simulink model "AccPed_DrvDemLead"  (R2016b)
settings: configuration reference "CodeGenConfigSet" (kept outside this file)
values from neighbouring files (symbols this model uses):
  ACCPED_OVRRUNRMP_SY = uint8(1)    [init_AccPed_DrvDemLead.m]    (also in init_AccPed_DrvDemLead_SIL.m)
  ACCPED_REVGEARMAP_SY = uint8(1)    [init_AccPed_DrvDemLead.m]    (also in init_AccPed_DrvDemLead_SIL.m)
  AccPed_rThresPrp_C = Calibration.Parameter    [init_AccPed_DrvDemLead.m]    (also in init_AccPed_DrvDemLead_SIL.m = Simulink.Parameter)
  AccPed_rZero_C = Calibration.Parameter    [init_AccPed_DrvDemLead.m]    (also in init_AccPed_DrvDemLead_SIL.m = Simulink.Parameter)
  AccPed_trqEngRev_MAP = Calibration.Parameter    [init_AccPed_DrvDemLead.m]    (also in init_AccPed_DrvDemLead_SIL.m = Simulink.Parameter)
  AccPed_trqEngRev_MAPX = Calibration.Parameter    [init_AccPed_DrvDemLead.m]    (also in init_AccPed_DrvDemLead_SIL.m = Simulink.Parameter)
  AccPed_trqEngRev_MAPY = Calibration.Parameter    [init_AccPed_DrvDemLead.m]    (also in init_AccPed_DrvDemLead_SIL.m = Simulink.Parameter)
  AccPed_trqPrp_MAP = Calibration.Parameter    [init_AccPed_DrvDemLead.m]    (also in init_AccPed_DrvDemLead_SIL.m = Simulink.Parameter)
  AccPed_trqPrp_MAPX = Calibration.Parameter    [init_AccPed_DrvDemLead.m]    (also in init_AccPed_DrvDemLead_SIL.m = Simulink.Parameter)
  AccPed_trqPrp_MAPY = Calibration.Parameter    [init_AccPed_DrvDemLead.m]    (also in init_AccPed_DrvDemLead_SIL.m = Simulink.Parameter)
  MoFDrDem_trqEng_MAP = Calibration.Parameter    [init_AccPed_DrvDemLead.m]    (also in init_AccPed_DrvDemLead_SIL.m = Simulink.Parameter)
  MoFDrDem_trqEng_MAPX = Calibration.Parameter    [init_AccPed_DrvDemLead.m]    (also in init_AccPed_DrvDemLead_SIL.m = Simulink.Parameter)
  MoFDrDem_trqEng_MAPY = Calibration.Parameter    [init_AccPed_DrvDemLead.m]    (also in init_AccPed_DrvDemLead_SIL.m = Simulink.Parameter)
  MSTSHFT_SY = uint8(0)    [init_AccPed_DrvDemLead.m]    (also in init_AccPed_DrvDemLead_SIL.m)
  SigTst_swtAccPedLead_C = Calibration.Parameter    [init_AccPed_DrvDemLead.m]    (also in init_AccPed_DrvDemLead_SIL.m = Simulink.Parameter)
  SigTst_trqAccPedLead_C = Calibration.Parameter    [init_AccPed_DrvDemLead.m]    (also in init_AccPed_DrvDemLead_SIL.m = Simulink.Parameter)
  TRQPRPHIGH_ZERO = int16(0)    [init_AccPed_DrvDemLead.m]    (also in init_AccPed_DrvDemLead_SIL.m)
undefined symbols (not defined in the file or in its folder): Switch_conv
settings Model: Creator=lenovo  LastModifiedBy=bianxuyin
settings ConfigSetRef: SourceLocation=Base Workspace

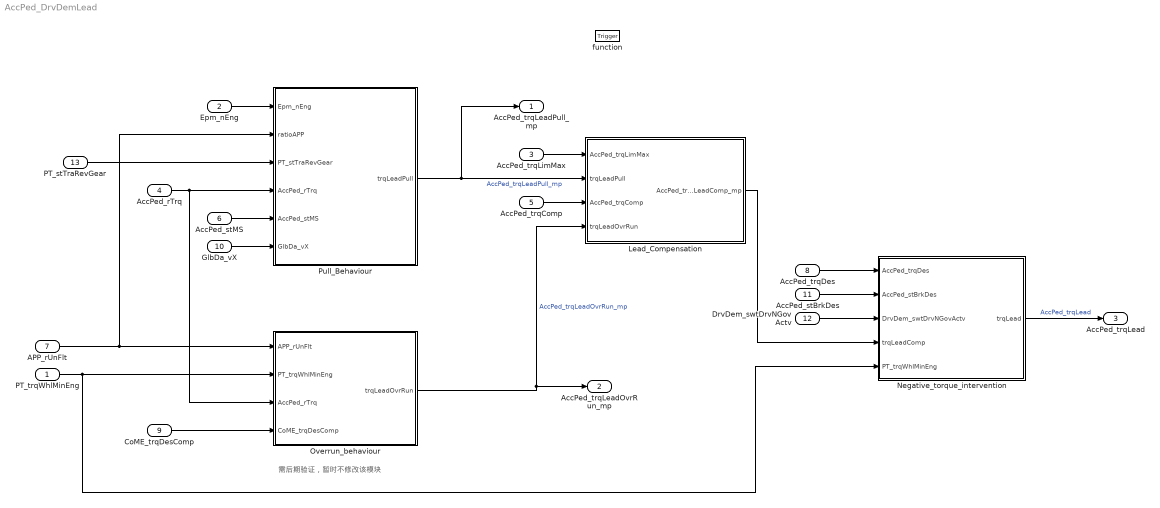
== system AccPed_DrvDemLead ==
  note: 需后期验证，暂时不修改该模块
  PT_trqWhlMinEng : Inport  Tag=Nm  Description=Minimum wheel torque from the engine  OutMin=-3000  OutMax=3000  OutDataTypeStr=Trq_Nm
  Epm_nEng : Inport  Tag=rpm  Description=Engine speed  Port=2  OutMin=0  OutMax=6000  OutDataTypeStr=EngSpeed_rpm
  AccPed_trqLimMax : Inport  Tag=Nm  Description=Maximum wheel torque in case of accelerator pedal error  Port=3  OutMin=-3000  OutMax=3000  OutDataTypeStr=Trq_Nm
  AccPed_rTrq : Inport  Description=Total drive train ratio of engine - wheel  Port=4  OutMin=-327  OutMax=327  OutDataTypeStr=TransRatio
  AccPed_trqComp : Inport  Tag=Nm  Description=Compensation torque of accelerator pedal  Port=5  OutMin=-3000  OutMax=3000  OutDataTypeStr=Trq_Nm
  AccPed_stMS : Inport  Description=Switch of the mastershift operation  Port=6  OutMin=0  OutMax=1  OutDataTypeStr=boolean
  APP_rUnFlt : Inport  Tag=%  Description=Unfiltered APP value  Port=7  OutMin=0  OutMax=100  OutDataTypeStr=Accpedal_rate
  AccPed_trqDes : Inport  Tag=Nm  Description=Driver torque value of propulsion after step limitation  Port=8  OutMin=-3000  OutMax=3000  OutDataTypeStr=Trq_Nm
  CoME_trqDesComp : Inport  Tag=Nm  Description=Application parameter for torque demand of mechanical co-ordinator  Port=9  OutMin=-3000  OutMax=3000  OutDataTypeStr=Trq_Nm
  GlbDa_vX : Inport  Tag=km/h  Description=Longitudinal vehicle speed (X-direction)  Port=10  OutMin=0  OutMax=250  OutDataTypeStr=VehSpeed_km_h
  AccPed_stBrkDes : Inport  Description=Application parameter for engine brake request  Port=11  OutMin=0  OutMax=255  OutDataTypeStr=State_uint8
  DrvDem_swtDrvNGovActv : Inport  Description=Switch to activate DrvDem  Port=12  OutDataTypeStr=Enum: Switch_conv
  PT_stTraRevGear : Inport  Description=Status if reverse gear is selected  Port=13  OutMin=0  OutMax=1  OutDataTypeStr=boolean
  function : TriggerPort  TriggerType=function-call  VariantControl=Variant
  Lead_Compensation : Subsystem
  Negative_torque_intervention : Subsystem
  Overrun_behaviour : Subsystem
  Pull_Behaviour : Subsystem
  AccPed_trqLeadPull_mp : Outport  Tag=Nm  Description=Driver command torque for pull component lead path  OutMin=-3000  OutMax=3000  OutDataTypeStr=Trq_Nm
  AccPed_trqLeadOvrRun_mp : Outport  Tag=Nm  Description=Driver command torque for overrun part lead path  Port=2  OutMin=-3000  OutMax=3000  OutDataTypeStr=Trq_Nm
  AccPed_trqLead : Outport  Tag=Nm  Description=Lead torque of accelerator pedal  Port=3  OutMin=-3000  OutMax=3000  OutDataTypeStr=Trq_Nm
  wires:
  AccPed_stBrkDes/1 -> Negative_torque_intervention/2(AccPed_stBrkDes)
  AccPed_trqDes/1 -> Negative_torque_intervention/1(AccPed_trqDes)
  GlbDa_vX/1 -> Pull_Behaviour/6(GlbDa_vX)
  CoME_trqDesComp/1 -> Overrun_behaviour/4(CoME_trqDesComp)
  Overrun_behaviour/1(trqLeadOvrRun) -> Lead_Compensation/4(trqLeadOvrRun), AccPed_trqLeadOvrRun_mp/1  "AccPed_trqLeadOvrRun_mp"
  APP_rUnFlt/1 -> Overrun_behaviour/1(APP_rUnFlt), Pull_Behaviour/2(ratioAPP)
  Pull_Behaviour/1(" trqLeadPull") -> Lead_Compensation/2(trqLeadPull), AccPed_trqLeadPull_mp/1  "AccPed_trqLeadPull_mp"
  Negative_torque_intervention/1(trqLead) -> AccPed_trqLead/1  "AccPed_trqLead"
  PT_trqWhlMinEng/1 -> Negative_torque_intervention/5(PT_trqWhlMinEng), Overrun_behaviour/2(PT_trqWhlMinEng)
  Epm_nEng/1 -> Pull_Behaviour/1(Epm_nEng)
  AccPed_rTrq/1 -> Overrun_behaviour/3(AccPed_rTrq), Pull_Behaviour/4(AccPed_rTrq)
  PT_stTraRevGear/1 -> Pull_Behaviour/3(PT_stTraRevGear)
  AccPed_stMS/1 -> Pull_Behaviour/5(AccPed_stMS)
  AccPed_trqLimMax/1 -> Lead_Compensation/1(AccPed_trqLimMax)
  AccPed_trqComp/1 -> Lead_Compensation/3(AccPed_trqComp)
  Lead_Compensation/1(AccPed_trqLeadComp_mp) -> Negative_torque_intervention/4(trqLeadComp)
  DrvDem_swtDrvNGovActv/1 -> Negative_torque_intervention/3(DrvDem_swtDrvNGovActv)

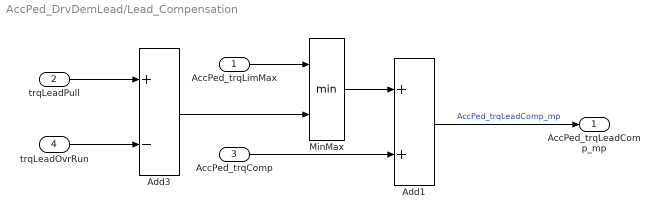
== system AccPed_DrvDemLead/Lead_Compensation ==
  AccPed_trqLimMax : Inport  Tag=Nm  Description=Maximum wheel torque in case of accelerator pedal error  OutMin=-3000  OutMax=3000  OutDataTypeStr=Trq_Nm
  trqLeadPull : Inport  Port=2
  AccPed_trqComp : Inport  Tag=Nm  Description=Compensation torque of accelerator pedal  Port=3  OutMin=-3000  OutMax=3000  OutDataTypeStr=Trq_Nm
  trqLeadOvrRun : Inport  Port=4
  Add1 : Sum  SaturateOnIntegerOverflow=on  InputSameDT=on
  Add3 : Sum  Inputs=+-  SaturateOnIntegerOverflow=on  InputSameDT=on
  MinMax : MinMax  Inputs=2  InputSameDT=on
  AccPed_trqLeadComp_mp : Outport
  wires:
  AccPed_trqLimMax/1 -> MinMax/1
  MinMax/1 -> Add1/1
  Add3/1 -> MinMax/2
  Add1/1 -> AccPed_trqLeadComp_mp/1  "AccPed_trqLeadComp_mp"
  AccPed_trqComp/1 -> Add1/2
  trqLeadPull/1 -> Add3/1
  trqLeadOvrRun/1 -> Add3/2

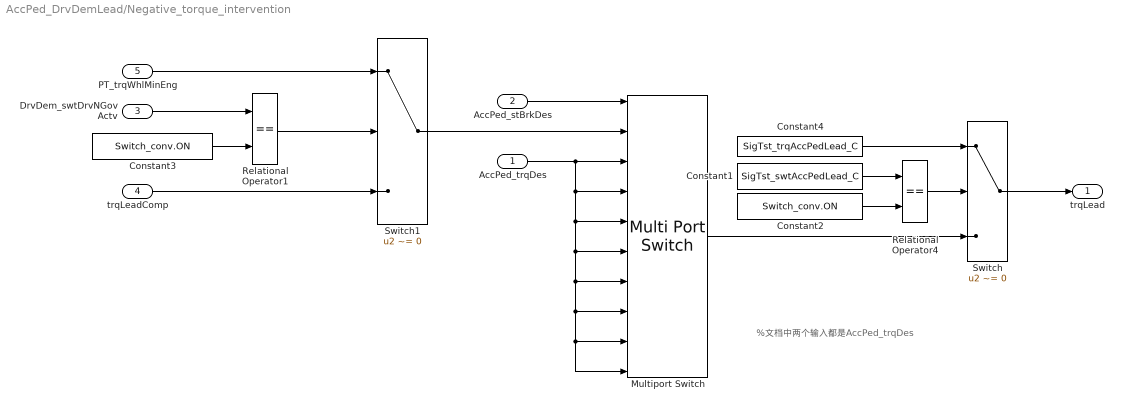
== system AccPed_DrvDemLead/Negative_torque_intervention ==
  note: %文档中两个输入都是AccPed_trqDes
  AccPed_trqDes : Inport  RequirementInfo={'other' 'APP_requirements.doc' '@Simulink_requirement_item_23' 'true' '振动过滤' '' } %GIDa_99f4ad60_2df5_4069_99f2_cc873ebc05b2
  AccPed_stBrkDes : Inport  RequirementInfo={'other' 'APP_requirements.doc' '@Simulink_requirement_item_23' 'true' '振动过滤' '' } %GIDa_759d7569_d091_4650_98e0_bc0acb76dd52  Port=2
  DrvDem_swtDrvNGovActv : Inport  Tag=-  Description=Switch to activate DrvDem  Port=3  OutDataTypeStr=Enum: Switch_conv
  trqLeadComp : Inport  RequirementInfo={'other' 'APP_requirements.doc' '@Simulink_requirement_item_23' 'true' '振动过滤' '' } %GIDa_a2b3fdec_2c90_459a_82d7_aebdd14e4d26  Port=4
  PT_trqWhlMinEng : Inport  RequirementInfo={'other' 'APP_requirements.doc' '@Simulink_requirement_item_23' 'true' '振动过滤' '' } %GIDa_b7683208_daa5_4048_8e69_80f1a98c329a  Port=5
  Constant1 : Constant  Value=SigTst_swtAccPedLead_C
  Constant2 : Constant  Value=Switch_conv.ON  OutDataTypeStr=Inherit: Inherit via back propagation
  Constant3 : Constant  Value=Switch_conv.ON  OutDataTypeStr=Inherit: Inherit via back propagation
  Constant4 : Constant  Value=SigTst_trqAccPedLead_C
  Multiport Switch : MultiPortSwitch  DataPortOrder=Specify indices  DataPortIndices={0,1,4,64,128,2,8,16,32}  InputSameDT=on
  Relational Operator1 : RelationalOperator  Operator===  OutDataTypeStr=boolean  RndMeth=Simplest  InputSameDT=on
  Relational Operator4 : RelationalOperator  Operator===  OutDataTypeStr=boolean  RndMeth=Simplest  InputSameDT=on
  Switch : Switch  Criteria=u2 ~= 0  InputSameDT=on
  Switch1 : Switch  Criteria=u2 ~= 0  InputSameDT=on
  trqLead : Outport
  wires:
  AccPed_stBrkDes/1 -> Multiport Switch/1
  Switch1/1 -> Multiport Switch/2
  AccPed_trqDes/1 -> Multiport Switch/3, Multiport Switch/4, Multiport Switch/5, Multiport Switch/6, Multiport Switch/7, Multiport Switch/8, Multiport Switch/9, Multiport Switch/10
  Multiport Switch/1 -> Switch/3
  Switch/1 -> trqLead/1
  Constant4/1 -> Switch/1
  Constant2/1 -> Relational Operator4/2
  Constant1/1 -> Relational Operator4/1
  Relational Operator4/1 -> Switch/2
  PT_trqWhlMinEng/1 -> Switch1/1
  Constant3/1 -> Relational Operator1/2
  Relational Operator1/1 -> Switch1/2
  DrvDem_swtDrvNGovActv/1 -> Relational Operator1/1
  trqLeadComp/1 -> Switch1/3

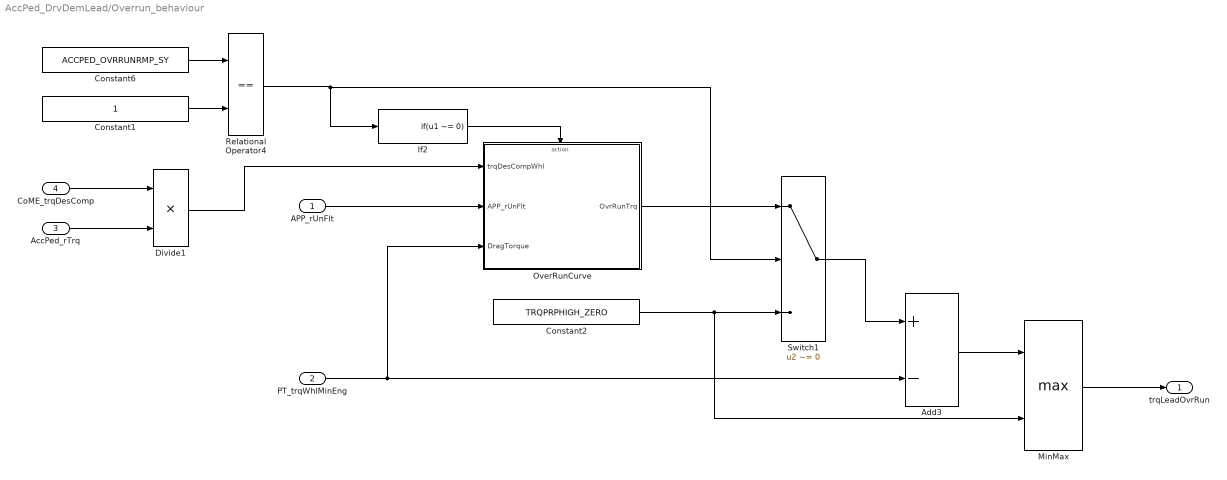
== system AccPed_DrvDemLead/Overrun_behaviour ==
  APP_rUnFlt : Inport  RequirementInfo={'other' 'APP_requirements.doc' '@Simulink_requirement_item_23' 'true' '振动过滤' '' } %GIDa_4c76d9da_ba24_4778_91f6_8f11bf935ee2
  PT_trqWhlMinEng : Inport  RequirementInfo={'other' 'APP_requirements.doc' '@Simulink_requirement_item_23' 'true' '振动过滤' '' } %GIDa_1da09a67_25cf_4f27_82fd_8354507ee43c  Port=2
  AccPed_rTrq : Inport  RequirementInfo={'other' 'APP_requirements.doc' '@Simulink_requirement_item_23' 'true' '振动过滤' '' } %GIDa_a0806bcb_2109_48e8_ade6_c61e01cb97cd  Port=3
  CoME_trqDesComp : Inport  Tag=Nm  Description=Application parameter for torque demand of mechanical co-ordinator  Port=4  OutMin=-3000  OutMax=3000  OutDataTypeStr=Trq_Nm
  Add3 : Sum  Inputs=+-  SaturateOnIntegerOverflow=on  InputSameDT=on
  Constant1 : Constant  RequirementInfo={'other' 'APP_requirements.doc' '@Simulink_requirement_item_25' 'true' '手动开关' '' } %GIDa_c1ebd30e_c358_4bd6_9f2e_8e035c9aac8e  OutDataTypeStr=Inherit: Inherit via back propagation
  Constant2 : Constant  RequirementInfo={'other' 'APP_requirements.doc' '@Simulink_requirement_item_25' 'true' '手动开关' '' } %GIDa_76cce100_95e7_4560_baf5_81e9c3f2f3d8  Value=TRQPRPHIGH_ZERO  OutDataTypeStr=Trq_Nm
  Constant6 : Constant  RequirementInfo={'other' 'APP_requirements.doc' '@Simulink_requirement_item_25' 'true' '手动开关' '' } %GIDa_71d7b391_d983_4443_a61c_479750307673  Value=ACCPED_OVRRUNRMP_SY
  Divide1 : Product  Inputs=**  OutDataTypeStr=Trq_Nm  SaturateOnIntegerOverflow=on
  If2 : If  IfExpression=u1 ~= 0  ShowElse=off
  MinMax : MinMax  Function=max  Inputs=2  InputSameDT=on
  OverRunCurve : Subsystem  TreatAsAtomicUnit=on
  Relational Operator4 : RelationalOperator  Operator===  OutDataTypeStr=boolean  RndMeth=Simplest  InputSameDT=on
  Switch1 : Switch  Criteria=u2 ~= 0  InputSameDT=on
  trqLeadOvrRun : Outport
  wires:
  Divide1/1 -> OverRunCurve/1(trqDesCompWhl)
  MinMax/1 -> trqLeadOvrRun/1
  Add3/1 -> MinMax/1
  Switch1/1 -> Add3/1
  OverRunCurve/1(OvrRunTrq) -> Switch1/1
  Constant2/1 -> Switch1/3, MinMax/2
  PT_trqWhlMinEng/1 -> Add3/2, OverRunCurve/3(DragTorque)
  APP_rUnFlt/1 -> OverRunCurve/2(APP_rUnFlt)
  Constant6/1 -> Relational Operator4/1
  Constant1/1 -> Relational Operator4/2
  Relational Operator4/1 -> Switch1/2, If2/1
  If2/1 -> OverRunCurve/Action
  CoME_trqDesComp/1 -> Divide1/1
  AccPed_rTrq/1 -> Divide1/2

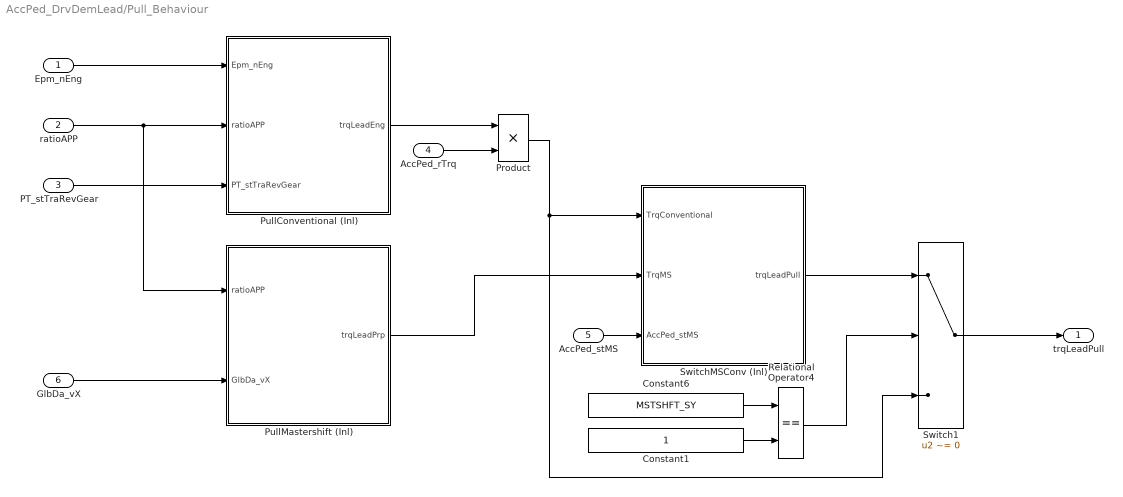
== system AccPed_DrvDemLead/Pull_Behaviour ==
  Epm_nEng : Inport  RequirementInfo={'other' 'APP_requirements.doc' '@Simulink_requirement_item_23' 'true' '振动过滤' '' } %GIDa_86b23878_46dc_4254_9b28_4f0f1ed1d376
  ratioAPP : Inport  RequirementInfo={'other' 'APP_requirements.doc' '@Simulink_requirement_item_23' 'true' '振动过滤' '' } %GIDa_4c76d9da_ba24_4778_91f6_8f11bf935ee2  Port=2
  PT_stTraRevGear : Inport  RequirementInfo={'other' 'APP_requirements.doc' '@Simulink_requirement_item_23' 'true' '振动过滤' '' } %GIDa_313c2354_c59f_427a_9e28_07fe0e6babea  Port=3
  AccPed_rTrq : Inport  RequirementInfo={'other' 'APP_requirements.doc' '@Simulink_requirement_item_23' 'true' '振动过滤' '' } %GIDa_8295bd3a_4d41_4b23_8842_c2b818804259  Port=4
  AccPed_stMS : Inport  RequirementInfo={'other' 'APP_requirements.doc' '@Simulink_requirement_item_23' 'true' '振动过滤' '' } %GIDa_866cc3c6_6713_4ba0_a34b_aeae0597c3e7  Port=5
  GlbDa_vX : Inport  RequirementInfo={'other' 'APP_requirements.doc' '@Simulink_requirement_item_23' 'true' '振动过滤' '' } %GIDa_56363f3f_5d85_4bed_afa1_e36614c2761f  Port=6
  Constant1 : Constant  RequirementInfo={'other' 'APP_requirements.doc' '@Simulink_requirement_item_25' 'true' '手动开关' '' } %GIDa_4cb955eb_cc9b_4184_bfb4_5ae11476adf1  OutDataTypeStr=Inherit: Inherit via back propagation
  Constant6 : Constant  RequirementInfo={'other' 'APP_requirements.doc' '@Simulink_requirement_item_25' 'true' '手动开关' '' } %GIDa_fb52ecf8_3c63_4a8c_95a9_cfdd3f88e07b  Value=MSTSHFT_SY
  Product : Product  OutDataTypeStr=Trq_Nm  SaturateOnIntegerOverflow=on
  PullConventional (Inl) : Subsystem  TreatAsAtomicUnit=on
  PullMastershift (Inl) : Subsystem  TreatAsAtomicUnit=on
  Relational Operator4 : RelationalOperator  Operator===  OutDataTypeStr=boolean  RndMeth=Simplest  InputSameDT=on
  Switch1 : Switch  Criteria=u2 ~= 0
  SwitchMSConv (Inl) : Subsystem  TreatAsAtomicUnit=on
  " trqLeadPull" : Outport
  wires:
  GlbDa_vX/1 -> PullMastershift (Inl)/2(GlbDa_vX)
  Switch1/1 -> " trqLeadPull"/1
  Relational Operator4/1 -> Switch1/2
  SwitchMSConv (Inl)/1(trqLeadPull) -> Switch1/1
  Constant6/1 -> Relational Operator4/1
  Constant1/1 -> Relational Operator4/2
  Product/1 -> SwitchMSConv (Inl)/1(TrqConventional), Switch1/3
  PullMastershift (Inl)/1(trqLeadPrp) -> SwitchMSConv (Inl)/2(TrqMS)
  AccPed_rTrq/1 -> Product/2
  PullConventional (Inl)/1(trqLeadEng) -> Product/1
  PT_stTraRevGear/1 -> PullConventional (Inl)/3(PT_stTraRevGear)
  ratioAPP/1 -> PullConventional (Inl)/2(ratioAPP), PullMastershift (Inl)/1(ratioAPP)
  Epm_nEng/1 -> PullConventional (Inl)/1(Epm_nEng)
  AccPed_stMS/1 -> SwitchMSConv (Inl)/3(AccPed_stMS)

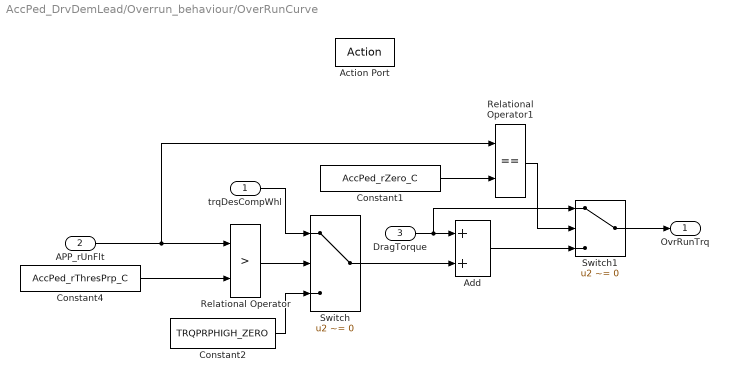
== system AccPed_DrvDemLead/Overrun_behaviour/OverRunCurve ==
  trqDesCompWhl : Inport
  APP_rUnFlt : Inport  Port=2
  DragTorque : Inport  Port=3
  Action Port : ActionPort  ActionType=then
  Add : Sum  SaturateOnIntegerOverflow=on
  Constant1 : Constant  Value=AccPed_rZero_C  VectorParams1D=off
  Constant2 : Constant  Value=TRQPRPHIGH_ZERO  OutDataTypeStr=Trq_Nm
  Constant4 : Constant  Value=AccPed_rThresPrp_C
  Relational Operator : RelationalOperator  Operator=>  OutDataTypeStr=boolean  RndMeth=Simplest
  Relational Operator1 : RelationalOperator  Operator===  OutDataTypeStr=boolean  RndMeth=Simplest
  Switch : Switch  Criteria=u2 ~= 0  InputSameDT=on
  Switch1 : Switch  Criteria=u2 ~= 0  InputSameDT=on
  OvrRunTrq : Outport
  wires:
  DragTorque/1 -> Add/1, Switch1/1
  Switch1/1 -> OvrRunTrq/1
  Constant1/1 -> Relational Operator1/2
  Relational Operator1/1 -> Switch1/2
  Constant2/1 -> Switch/3
  Switch/1 -> Add/2
  Relational Operator/1 -> Switch/2
  APP_rUnFlt/1 -> Relational Operator/1, Relational Operator1/1
  Constant4/1 -> Relational Operator/2
  trqDesCompWhl/1 -> Switch/1
  Add/1 -> Switch1/3

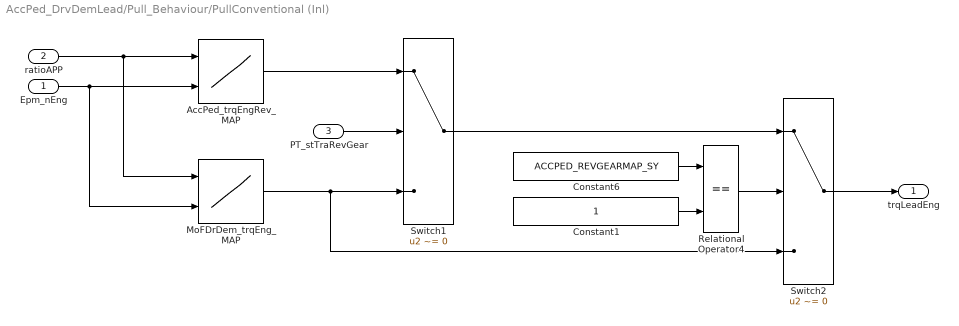
== system AccPed_DrvDemLead/Pull_Behaviour/PullConventional (Inl) ==
  Epm_nEng : Inport  RequirementInfo={'other' 'APP_requirements.doc' '@Simulink_requirement_item_23' 'true' '振动过滤' '' } %GIDa_cdbf5cb3_02b2_4bec_885e_3f105a7bb510
  ratioAPP : Inport  RequirementInfo={'other' 'APP_requirements.doc' '@Simulink_requirement_item_23' 'true' '振动过滤' '' } %GIDa_e14b1247_bfdb_4616_8b10_4d89c5371701  Port=2
  PT_stTraRevGear : Inport  RequirementInfo={'other' 'APP_requirements.doc' '@Simulink_requirement_item_23' 'true' '振动过滤' '' } %GIDa_32104aab_869e_45e1_aa0f_2090fc18c91a  Port=3
  AccPed_trqEngRev_MAP : Lookup_n-D  BreakpointsForDimension1=AccPed_trqEngRev_MAPY  BreakpointsForDimension2=AccPed_trqEngRev_MAPX  IndexSearchMethod=Linear search  BeginIndexSearchUsingPreviousIndexResult=on  Table=AccPed_trqEngRev_MAP  ExtrapMethod=Clip  UseLastTableValue=on  InternalRulePriority=Speed  OutDataTypeStr=Inherit: Inherit via back propagation  RndMeth=Simplest  SaturateOnIntegerOverflow=on
  Constant1 : Constant  RequirementInfo={'other' 'APP_requirements.doc' '@Simulink_requirement_item_25' 'true' '手动开关' '' } %GIDa_60fba1eb_beb4_46b4_b1a1_41c2fbb77e62  OutDataTypeStr=Inherit: Inherit via back propagation
  Constant6 : Constant  RequirementInfo={'other' 'APP_requirements.doc' '@Simulink_requirement_item_25' 'true' '手动开关' '' } %GIDa_405aa919_fe57_4ba9_beda_0486a3185c1e  Value=ACCPED_REVGEARMAP_SY
  MoFDrDem_trqEng_MAP : Lookup_n-D  BreakpointsForDimension1=MoFDrDem_trqEng_MAPY  BreakpointsForDimension2=MoFDrDem_trqEng_MAPX  IndexSearchMethod=Linear search  BeginIndexSearchUsingPreviousIndexResult=on  Table=MoFDrDem_trqEng_MAP  ExtrapMethod=Clip  UseLastTableValue=on  InternalRulePriority=Speed  OutDataTypeStr=Inherit: Inherit via back propagation  RndMeth=Simplest  SaturateOnIntegerOverflow=on
  Relational Operator4 : RelationalOperator  Operator===  OutDataTypeStr=boolean  RndMeth=Simplest  InputSameDT=on
  Switch1 : Switch  Criteria=u2 ~= 0  InputSameDT=on
  Switch2 : Switch  Criteria=u2 ~= 0  InputSameDT=on
  trqLeadEng : Outport
  wires:
  Switch2/1 -> trqLeadEng/1
  Switch1/1 -> Switch2/1
  Relational Operator4/1 -> Switch2/2
  Constant6/1 -> Relational Operator4/1
  Constant1/1 -> Relational Operator4/2
  MoFDrDem_trqEng_MAP/1 -> Switch2/3, Switch1/3
  AccPed_trqEngRev_MAP/1 -> Switch1/1
  PT_stTraRevGear/1 -> Switch1/2
  Epm_nEng/1 -> AccPed_trqEngRev_MAP/2, MoFDrDem_trqEng_MAP/2
  ratioAPP/1 -> AccPed_trqEngRev_MAP/1, MoFDrDem_trqEng_MAP/1

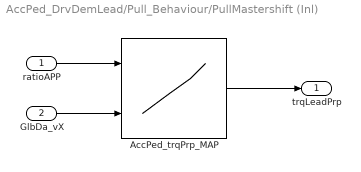
== system AccPed_DrvDemLead/Pull_Behaviour/PullMastershift (Inl) ==
  ratioAPP : Inport
  GlbDa_vX : Inport  Port=2
  AccPed_trqPrp_MAP : Lookup_n-D  BreakpointsForDimension1=AccPed_trqPrp_MAPY  BreakpointsForDimension2=AccPed_trqPrp_MAPX  IndexSearchMethod=Linear search  BeginIndexSearchUsingPreviousIndexResult=on  Table=AccPed_trqPrp_MAP  ExtrapMethod=Clip  UseLastTableValue=on  InternalRulePriority=Speed  OutDataTypeStr=Inherit: Inherit via back propagation  SaturateOnIntegerOverflow=on
  trqLeadPrp : Outport
  wires:
  GlbDa_vX/1 -> AccPed_trqPrp_MAP/2
  ratioAPP/1 -> AccPed_trqPrp_MAP/1
  AccPed_trqPrp_MAP/1 -> trqLeadPrp/1

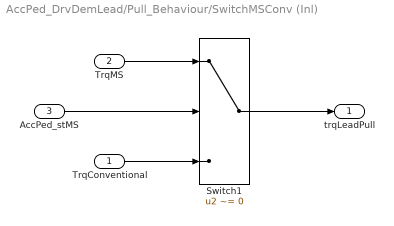
== system AccPed_DrvDemLead/Pull_Behaviour/SwitchMSConv (Inl) ==
  TrqConventional : Inport  RequirementInfo={'other' 'APP_requirements.doc' '@Simulink_requirement_item_23' 'true' '振动过滤' '' } %GIDa_e14b1247_bfdb_4616_8b10_4d89c5371701
  TrqMS : Inport  RequirementInfo={'other' 'APP_requirements.doc' '@Simulink_requirement_item_23' 'true' '振动过滤' '' } %GIDa_ea405ce8_8a78_4f53_80fe_9d47b047bbf5  Port=2
  AccPed_stMS : Inport  RequirementInfo={'other' 'APP_requirements.doc' '@Simulink_requirement_item_23' 'true' '振动过滤' '' } %GIDa_ce622dc4_d714_4310_830e_668fe57966be  Port=3
  Switch1 : Switch  Criteria=u2 ~= 0  InputSameDT=on
  trqLeadPull : Outport
  wires:
  Switch1/1 -> trqLeadPull/1
  TrqConventional/1 -> Switch1/3
  TrqMS/1 -> Switch1/1
  AccPed_stMS/1 -> Switch1/2
